simulink model "Synchr"  (Simulink 4.00)
settings: Solver=ode23tb  StartTime=0.0  StopTime=0.1
InitFcn:
  | powericon('psbinitsys',bdroot);
libraries: powerlib_extras x3, powerlib2 x3
settings Model: LastModifiedBy=ieao  SaveTime=off  SaveOutput=off  LimitDataPoints=off  BlockReductionOpt=off

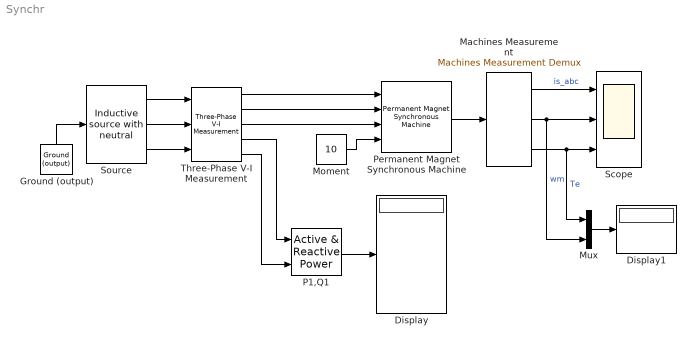
== system Synchr ==
  " Source" : powerlib_extras/Three-Phase Library/Inductive source with neutral  V=310  Phi=0  F=50  R=0.724  L=0
  Display : Display
      settings: Format=short
  Display1 : Display
      settings: Format=short
  Ground (output) : powerlib2/Connectors/Ground (output)  Tag=PoWeRsYsTeMbLoCk  Orientation=up  PSBOutputType=1
  Machines Measurement : powerlib2/Machines/Machines Measurement Demux  machType=Permanent magnet synchronous  ssm1=on  ssm2=off  ssm3=on  ssm4=off  ssm5=on  ssm6=off  sm1=on  sm2=on  sm3=on  sm4=on  sm5=on  sm6=on  sm7=on  sm8=on  sm9=on  sm10=on  sm11=on  asm1=on  asm2=on  asm3=on  asm4=on  asm5=on  asm6=on  asm7=on  asm8=on  asm9=on  asm10=on  asm11=on  pmsm1=on  pmsm2=off  pmsm3=off  pmsm4=on  pmsm5=off  pmsm6=on  lastType=1
  Moment : Constant  Value=10
  Mux : Mux  Inputs=2
  P1,Q1 : powerlib_extras/Measurements/Active & Reactive Power  f1=50
  Permanent Magnet Synchronous Machine : powerlib2/Machines/Permanent Magnet Synchronous Machine  Tag=PoWeRsYsTeMbLoCk  x1=2.8  x2=[8.5e-3, 2.5e-3]  x3=1  x4="[ 0.8e-3, 0,  4 ]"  PSBOutputType=0
  Scope : Scope  NumInputPorts=3
      settings: TimeRange=auto  YMin=-75~-50~-40  YMax=100~300~40  SaveToWorkspace=off  SaveName=ScopeData  MaxDataPoints=5000
  Three-Phase V-I Measurement : powerlib_extras/Measurements/Three-Phase V-I Measurement  phaseurs=off  Vpu=off  Vbase=500e3  Ppu=off  Pbase=100e6
  wires:
  Permanent Magnet Synchronous Machine/1 -> Machines Measurement/1
  Three-Phase V-I Measurement/1 -> Permanent Magnet Synchronous Machine/1
  Three-Phase V-I Measurement/2 -> Permanent Magnet Synchronous Machine/2
  Three-Phase V-I Measurement/3 -> Permanent Magnet Synchronous Machine/3
  Moment/1 -> Permanent Magnet Synchronous Machine/4
  Machines Measurement/2 -> Scope/2, Mux/2  "wm"
  Three-Phase V-I Measurement/4 -> P1,Q1/1
  Three-Phase V-I Measurement/5 -> P1,Q1/2
  " Source"/1 -> Three-Phase V-I Measurement/1
  P1,Q1/1 -> Display/1
  Ground (output)/1 -> " Source"/1
  " Source"/2 -> Three-Phase V-I Measurement/2
  " Source"/3 -> Three-Phase V-I Measurement/3
  Machines Measurement/1 -> Scope/1  "is_abc"
  Mux/1 -> Display1/1
  Machines Measurement/3 -> Mux/1, Scope/3  "Te"
